simulink model "ControlBA"  (R2023b)
settings: Solver=FixedStepDiscrete  StartTime=0.0  StopTime=inf  FixedStep=0.01  RelTol=1e-3  EnableMultiTasking=on
settings Model: ExtModeTrigDuration=2  Creator=Antonio  LastModifiedBy=Antonio
settings OptimizationCC: EnhancedBackFolding=on  PassReuseOutputArgsAs=Individual arguments  ZeroExternalMemoryAtStartup=off  ZeroInternalMemoryAtStartup=off  MaxStackSize=64  OptimizeBlockOrder=speed  DifferentSizesBufferReuse=on  OptimizationCustomize=off  EfficientTunableParamExpr=on
settings DebuggingCC: ParameterTunabilityLossMsg=error
settings HardwareCC: ProdBitPerInt=16  ProdBitPerPointer=16  ProdBitPerSizeT=16  ProdBitPerPtrDiffT=16  ProdLargestAtomicFloat=None  ProdWordSize=8  ProdHWDeviceType=Atmel->AVR
settings SFSimCC: MATLABDynamicMemAlloc=off
settings RTWCC: Description=Embedded Coder  SystemTargetFile=ert.tlc  HardwareBoard=Arduino Mega 2560  TemplateMakefile=ert_default_tmf  Toolchain=Arduino AVR  BuildConfiguration=Faster Runs
settings CodeAppCC: ForceParamTrailComments=on  IgnoreCustomStorageClasses=off  OperatorAnnotations=on  SimulinkDataObjDesc=on  SFDataObjDesc=on  InsertBlockDesc=on
settings ERTTargetCC: SupportContinuousTime=on  SupportVariableSizeSignals=on  ExtModeTransport=3  ExtModeStaticAlloc=on  ExtModeAutomaticAllocSize=off  ExtModeStaticAllocSize=2048  ExtModeMexFile=ext_xcp  ExtModeIntrfLevel=Level2 - Open

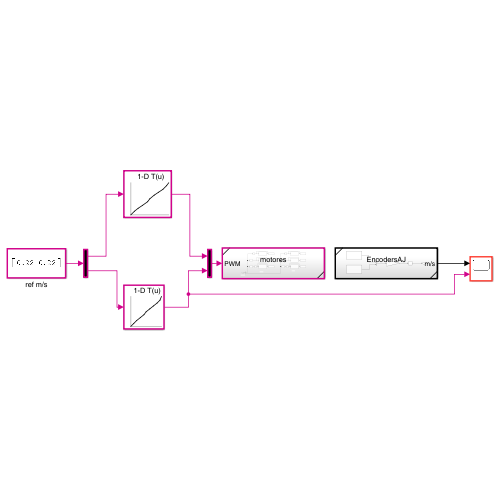
[thumbnail: Simulink's stored preview of the top-level diagram]
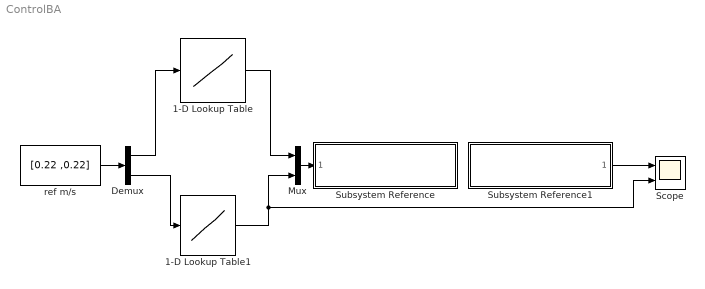
== system ControlBA ==
  1-D Lookup Table : Lookup_n-D  NumberOfTableDimensions=1  BreakpointsForDimension1=[-0.38158318400383 -0.309403449296951 -0.237214490771294 -0.154694348573685 -0.0515652559697628 0 0.0825028643012047 0.175317093729973 0.257832050323486 0.330025285482407 0.371277689933777]  Table=[-255 -200 -150 -100 -50 0 50 100 150 200 255]  InternalRulePriority=Speed  RndMeth=Simplest
  1-D Lookup Table1 : Lookup_n-D  NumberOfTableDimensions=1  BreakpointsForDimension1=[-0.38158318400383 -0.309403449296951 -0.237214490771294 -0.154694348573685 -0.0515652559697628 0 0.0825028643012047 0.175317093729973 0.257832050323486 0.330025285482407 0.371277689933777]  Table=[-255 -200 -150 -100 -50 0 50 100 150 200 255]  InternalRulePriority=Speed  RndMeth=Simplest
  Demux : Demux  Outputs=2
  Mux : Mux  Inputs=2
  Scope : Scope  NumInputPorts=2
  Subsystem Reference : Subsystem  ReferencedSubsystem=motores
  Subsystem Reference1 : Subsystem  ReferencedSubsystem=EncodersAJ
  ref m/s : Constant  Value=[0.22 ,0.22]
  wires:
  Mux/1 -> Subsystem Reference/1
  Subsystem Reference1/1 -> Scope/1
  ref m/s/1 -> Demux/1
  Demux/1 -> 1-D Lookup Table/1
  1-D Lookup Table/1 -> Mux/1
  1-D Lookup Table1/1 -> Scope/2, Mux/2
  Demux/2 -> 1-D Lookup Table1/1
